simulink model "Propuesta_modelo_LIM"  (R2022b)
settings: Solver=VariableStepAuto  StartTime=0.0  StopTime=10.0  RelTol=1e-3
undefined symbols (not defined in the file or in its folder): mass, pole_length, Ref_velocity
libraries: slpidlib x2
settings Model: Creator=Javier  LastModifiedBy=Javier
settings DebuggingCC: UnconnectedInputMsg=warning  UnconnectedOutputMsg=warning  UnconnectedLineMsg=warning
settings ModelReferenceCC: EnableRefExpFcnMdlSchedulingChecks=on
settings RTWCC: DLArmComputeVersion=19.05

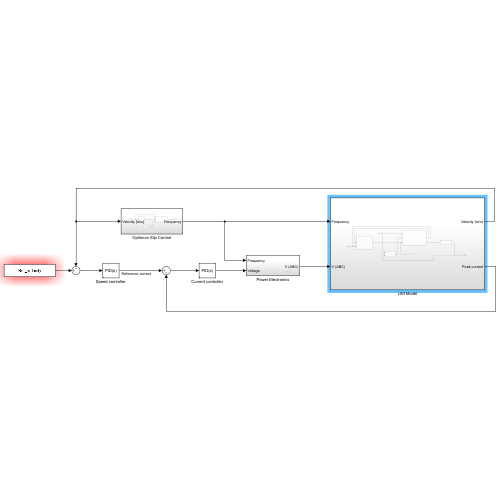
[thumbnail: Simulink's stored preview of the top-level diagram]
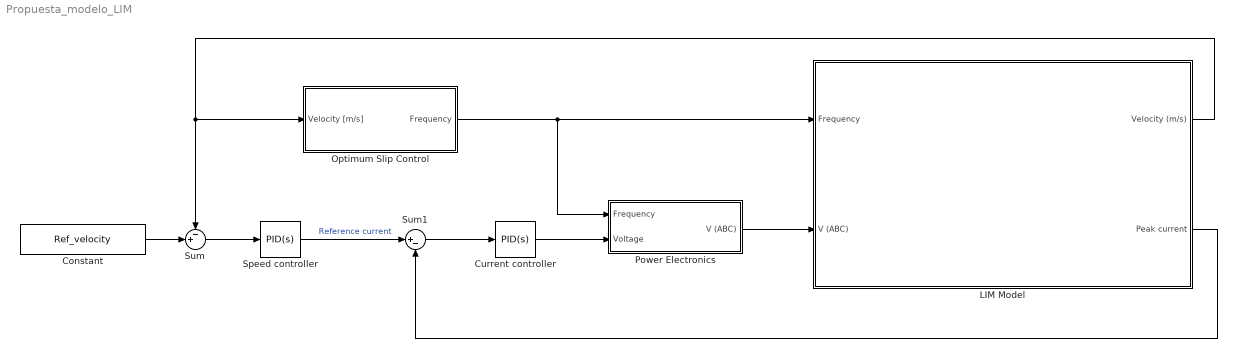
== system Propuesta_modelo_LIM ==
  Constant : Constant  Value=Ref_velocity
  Current controller : slpidlib/PID Controller  Controller=PID  Form=Parallel  TimeDomain=Continuous-time  UseExternalTs=off  SampleTime=-1  IntegratorMethod=Forward Euler  FilterMethod=Forward Euler  ControllerParametersSource=internal  P=1  I=1  UseKiTs=off  D=0  N=100  UseFilter=on  TunerSelectOption=Transfer Function Based (PID Tuner App)  InitialConditionSource=internal  InitialConditionForIntegrator=0  InitialConditionForFilter=0  DifferentiatorICPrevScaledInput=0  ExternalReset=none  TrackingMode=off  Kt=1  LimitOutput=off  SatLimitsSource=internal  UpperSaturationLimit=inf  LowerSaturationLimit=-inf  LinearizeAsGain=on  AntiWindupMode=none  Kb=1  LimitIntegrator=off  UpperIntegratorSaturationLimit=inf  LowerIntegratorSaturationLimit=-inf  POutMin=[]  POutMax=[]  IOutMin=[]  IOutMax=[]  DOutMin=[]  DOutMax=[]  NOutMin=[]  NOutMax=[]  SumOutMin=[]  SumOutMax=[]  SaturationOutMin=[]  SaturationOutMax=[]  PParamMin=[]  PParamMax=[]  IParamMin=[]  IParamMax=[]  DParamMin=[]  DParamMax=[]  NParamMin=[]  NParamMax=[]  KbParamMin=[]  KbParamMax=[]  KtParamMin=[]  KtParamMax=[]  KbOutMin=[]  KbOutMax=[]  KtOutMin=[]  KtOutMax=[]  IntegratorOutMin=[]  IntegratorOutMax=[]  FilterOutMin=[]  FilterOutMax=[]  SumI1OutMin=[]  SumI1OutMax=[]  SumI2OutMin=[]  SumI2OutMax=[]  SumI3OutMin=[]  SumI3OutMax=[]  SumI4OutMin=[]  SumI4OutMax=[]  SumDOutMin=[]  SumDOutMax=[]  DifferentiatorOutMin=[]  DifferentiatorOutMax=[]  FilterDiffOutCoefMin=[]  FilterDiffOutCoefMax=[]  ReciprocalOutMin=[]  ReciprocalOutMax=[]  SumDenOutMin=[]  SumDenOutMax=[]  SumNumOutMin=[]  SumNumOutMax=[]  DivideOutMin=[]  DivideOutMax=[]  UdiffTsProdOutMin=[]  UdiffTsProdOutMax=[]  NTsProdOutMin=[]  NTsProdOutMax=[]  UintegralTsProdOutMin=[]  UintegralTsProdOutMax=[]  UngainTsProdOutMin=[]  UngainTsProdOutMax=[]  ClampingZeroOutDataTypeStr=Inherit: Inherit via back propagation  ClampingZeroOutMin=[]  ClampingZeroOutMax=[]  FilterDenConstantOutDataTypeStr=Inherit: Inherit via back propagation  FilterDenConstantOutMin=[]  FilterDenConstantOutMax=[]  PCopyOutDataTypeStr=Inherit: Inherit via back propagation  PCopyOutMin=[]  PCopyOutMax=[]  NCopyOutDataTypeStr=Inherit: Inherit via back propagation  NCopyOutMin=[]  NCopyOutMax=[]  IntegratorContinuousStateAttributes=''  IntegratorStateMustResolveToSignalObject=off  IntegratorRTWStateStorageClass=Auto  FilterContinuousStateAttributes=''  FilterStateMustResolveToSignalObject=off  FilterRTWStateStorageClass=Auto  ParallelPVariant=InternalParameters  IdealPVariant=Disabled  IVariant=InternalParameters  DVariant=InternalParameters  IntegratorVariant=Continuous  SatVariant=Disabled  AWVariant=Passthrough  PCopyVariant=Disabled  TRVariant=Disabled  FdbkBlocksVariant=Forward  IdealPFdbkVariant=Disabled  SatFdbkVariant=Disabled  DerivativeFilterVariant=ContFilter  NVariant=InternalParameters  NCopyVariant=Disabled  FilterICVariant=InternalICsFilter  IntegratorICVariant=InternalICs  ExternalResetVariant=Disabled  TRSumVariant=Passthrough  SumFdbkVariant=Disabled  SumVariant=Sum_PID  TsampFilterVariant=InternalTs  TsampNgainVariant=Passthrough  TsampIntegralVariant=Passthrough  ExternalSaturationOutDataTypeStr=Inherit: Same as second input
  LIM Model : Subsystem
  Optimum Slip Control : Subsystem
  Power Electronics : Subsystem
  Speed controller : slpidlib/PID Controller  Controller=PID  Form=Parallel  TimeDomain=Continuous-time  UseExternalTs=off  SampleTime=-1  IntegratorMethod=Forward Euler  FilterMethod=Forward Euler  ControllerParametersSource=internal  P=1  I=1  UseKiTs=off  D=0  N=100  UseFilter=on  TunerSelectOption=Transfer Function Based (PID Tuner App)  InitialConditionSource=internal  InitialConditionForIntegrator=0  InitialConditionForFilter=0  DifferentiatorICPrevScaledInput=0  ExternalReset=none  TrackingMode=off  Kt=1  LimitOutput=off  SatLimitsSource=internal  UpperSaturationLimit=inf  LowerSaturationLimit=-inf  LinearizeAsGain=on  AntiWindupMode=none  Kb=1  LimitIntegrator=off  UpperIntegratorSaturationLimit=inf  LowerIntegratorSaturationLimit=-inf  POutMin=[]  POutMax=[]  IOutMin=[]  IOutMax=[]  DOutMin=[]  DOutMax=[]  NOutMin=[]  NOutMax=[]  SumOutMin=[]  SumOutMax=[]  SaturationOutMin=[]  SaturationOutMax=[]  PParamMin=[]  PParamMax=[]  IParamMin=[]  IParamMax=[]  DParamMin=[]  DParamMax=[]  NParamMin=[]  NParamMax=[]  KbParamMin=[]  KbParamMax=[]  KtParamMin=[]  KtParamMax=[]  KbOutMin=[]  KbOutMax=[]  KtOutMin=[]  KtOutMax=[]  IntegratorOutMin=[]  IntegratorOutMax=[]  FilterOutMin=[]  FilterOutMax=[]  SumI1OutMin=[]  SumI1OutMax=[]  SumI2OutMin=[]  SumI2OutMax=[]  SumI3OutMin=[]  SumI3OutMax=[]  SumI4OutMin=[]  SumI4OutMax=[]  SumDOutMin=[]  SumDOutMax=[]  DifferentiatorOutMin=[]  DifferentiatorOutMax=[]  FilterDiffOutCoefMin=[]  FilterDiffOutCoefMax=[]  ReciprocalOutMin=[]  ReciprocalOutMax=[]  SumDenOutMin=[]  SumDenOutMax=[]  SumNumOutMin=[]  SumNumOutMax=[]  DivideOutMin=[]  DivideOutMax=[]  UdiffTsProdOutMin=[]  UdiffTsProdOutMax=[]  NTsProdOutMin=[]  NTsProdOutMax=[]  UintegralTsProdOutMin=[]  UintegralTsProdOutMax=[]  UngainTsProdOutMin=[]  UngainTsProdOutMax=[]  ClampingZeroOutDataTypeStr=Inherit: Inherit via back propagation  ClampingZeroOutMin=[]  ClampingZeroOutMax=[]  FilterDenConstantOutDataTypeStr=Inherit: Inherit via back propagation  FilterDenConstantOutMin=[]  FilterDenConstantOutMax=[]  PCopyOutDataTypeStr=Inherit: Inherit via back propagation  PCopyOutMin=[]  PCopyOutMax=[]  NCopyOutDataTypeStr=Inherit: Inherit via back propagation  NCopyOutMin=[]  NCopyOutMax=[]  IntegratorContinuousStateAttributes=''  IntegratorStateMustResolveToSignalObject=off  IntegratorRTWStateStorageClass=Auto  FilterContinuousStateAttributes=''  FilterStateMustResolveToSignalObject=off  FilterRTWStateStorageClass=Auto  ParallelPVariant=InternalParameters  IdealPVariant=Disabled  IVariant=InternalParameters  DVariant=InternalParameters  IntegratorVariant=Continuous  SatVariant=Disabled  AWVariant=Passthrough  PCopyVariant=Disabled  TRVariant=Disabled  FdbkBlocksVariant=Forward  IdealPFdbkVariant=Disabled  SatFdbkVariant=Disabled  DerivativeFilterVariant=ContFilter  NVariant=InternalParameters  NCopyVariant=Disabled  FilterICVariant=InternalICsFilter  IntegratorICVariant=InternalICs  ExternalResetVariant=Disabled  TRSumVariant=Passthrough  SumFdbkVariant=Disabled  SumVariant=Sum_PID  TsampFilterVariant=InternalTs  TsampNgainVariant=Passthrough  TsampIntegralVariant=Passthrough  ExternalSaturationOutDataTypeStr=Inherit: Same as second input
  Sum : Sum  Inputs=-+|
  Sum1 : Sum  Inputs=|+-
  wires:
  Sum/1 -> Speed controller/1
  LIM Model/1(Velocity (m/s)) -> Sum/1, Optimum Slip Control/1(Velocity [m/s])
  Speed controller/1 -> Sum1/1  "Reference current"
  Current controller/1 -> Power Electronics/2(Voltage)
  Sum1/1 -> Current controller/1
  LIM Model/2(Peak current) -> Sum1/2
  Optimum Slip Control/1(Frequency) -> Power Electronics/1(Frequency), LIM Model/1(Frequency)
  Constant/1 -> Sum/2
  Power Electronics/1(V (ABC)) -> LIM Model/2(V (ABC))

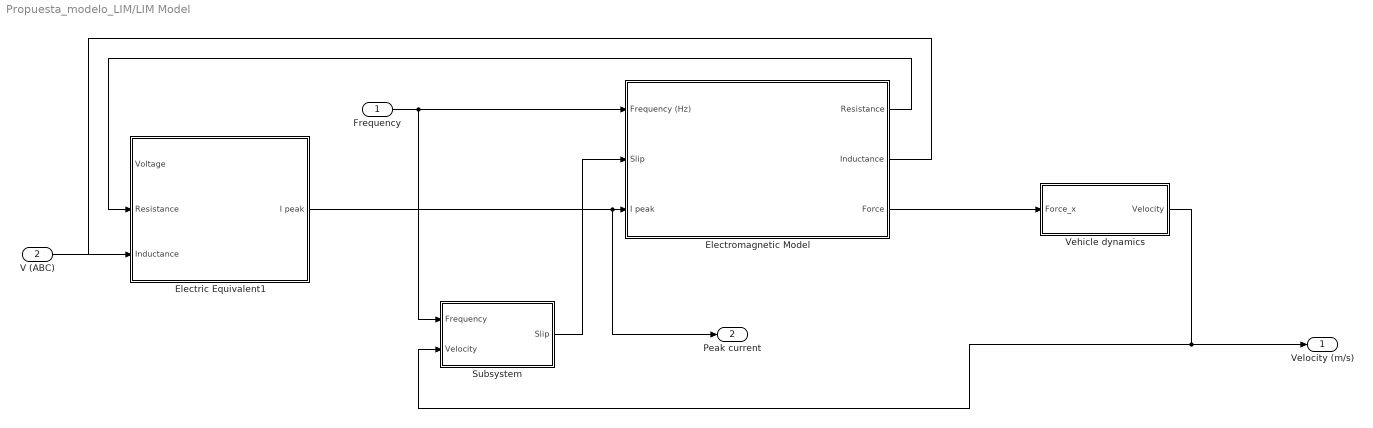
== system Propuesta_modelo_LIM/LIM Model ==
  Frequency : Inport
  V (ABC) : Inport  Port=2
  Electric Equivalent1 : Subsystem
  Electromagnetic Model : Subsystem
  Subsystem : Subsystem
  Vehicle dynamics : Subsystem
  Velocity (m/s) : Outport
  Peak current : Outport  Port=2
  wires:
  Subsystem/1(Slip) -> Electromagnetic Model/2(Slip)
  Vehicle dynamics/1(Velocity) -> Subsystem/2(Velocity), Velocity (m/s)/1
  Electric Equivalent1/1(I peak) -> Peak current/1, Electromagnetic Model/3(I peak)
  Electromagnetic Model/1(Resistance) -> Electric Equivalent1/2(Resistance)
  Electromagnetic Model/2(Inductance) -> Electric Equivalent1/3(Inductance)
  V (ABC)/1 -> ?
  Frequency/1 -> Electromagnetic Model/1(Frequency (Hz)), Subsystem/1(Frequency)
  Electromagnetic Model/3(Force) -> Vehicle dynamics/1(Force_x)

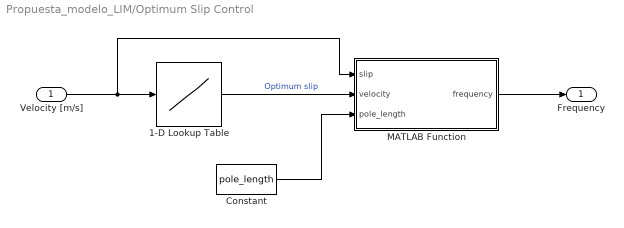
== system Propuesta_modelo_LIM/Optimum Slip Control ==
  Velocity [m/s] : Inport
  1-D Lookup Table : Lookup_n-D  NumberOfTableDimensions=1  BreakpointsForDimension1=[-5:5]  Table=tanh([-5:5])  InternalRulePriority=Speed  RndMeth=Simplest
  Constant : Constant  Value=pole_length
  MATLAB Function : MATLAB Function  TreatAsAtomicUnit=on
  Frequency : Outport
  wires:
  Velocity [m/s]/1 -> MATLAB Function/1(slip), 1-D Lookup Table/1
  1-D Lookup Table/1 -> MATLAB Function/2(velocity)  "Optimum slip"
  MATLAB Function/1(frequency) -> Frequency/1
  Constant/1 -> MATLAB Function/3(pole_length)

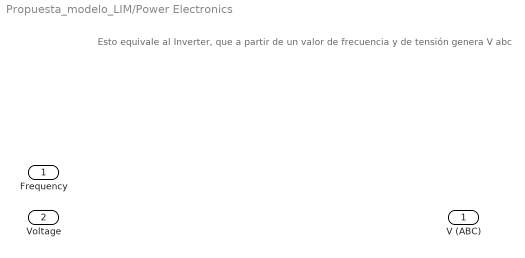
== system Propuesta_modelo_LIM/Power Electronics ==
  note: Esto equivale al Inverter, que a partir de un valor de frecuencia y de tensión genera V abc
  Frequency : Inport
  Voltage : Inport  Port=2
  V (ABC) : Outport

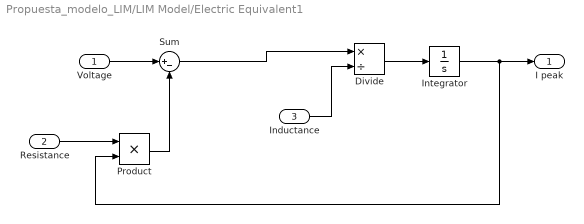
== system Propuesta_modelo_LIM/LIM Model/Electric Equivalent1 ==
  Voltage : Inport
  Resistance : Inport  Port=2
  Inductance : Inport  Port=3
  Divide : Product  Inputs=*/
  Integrator : Integrator
  Product : Product
  Sum : Sum  Inputs=|+-
  I peak : Outport
  wires:
  Voltage/1 -> Sum/1
  Integrator/1 -> Product/2, I peak/1
  Resistance/1 -> Product/1
  Product/1 -> Sum/2
  Divide/1 -> Integrator/1
  Sum/1 -> Divide/1
  Inductance/1 -> Divide/2

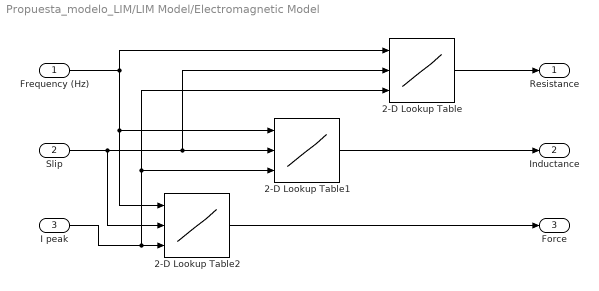
== system Propuesta_modelo_LIM/LIM Model/Electromagnetic Model ==
  Frequency (Hz) : Inport
  Slip : Inport  Port=2
  I peak : Inport  Port=3
  2-D Lookup Table : Lookup_n-D  NumberOfTableDimensions=3  BreakpointsForDimension1=[1:3]  BreakpointsForDimension2=[1:3]  InternalRulePriority=Speed  RndMeth=Simplest
      settings: InputPortMap=u0,u1,u2
  2-D Lookup Table1 : Lookup_n-D  NumberOfTableDimensions=3  BreakpointsForDimension1=[1:3]  BreakpointsForDimension2=[1:3]  InternalRulePriority=Speed  RndMeth=Simplest
      settings: InputPortMap=u0,u1,u2
  2-D Lookup Table2 : Lookup_n-D  NumberOfTableDimensions=3  BreakpointsForDimension1=[1:3]  BreakpointsForDimension2=[1:3]  InternalRulePriority=Speed  RndMeth=Simplest
      settings: InputPortMap=u0,u1,u2
  Resistance : Outport
  Inductance : Outport  Port=2
  Force : Outport  Port=3
  wires:
  2-D Lookup Table/1 -> Resistance/1
  2-D Lookup Table1/1 -> Inductance/1
  2-D Lookup Table2/1 -> Force/1
  I peak/1 -> 2-D Lookup Table1/3, 2-D Lookup Table/3, 2-D Lookup Table2/3
  Slip/1 -> 2-D Lookup Table2/2, 2-D Lookup Table/2, 2-D Lookup Table1/2
  Frequency (Hz)/1 -> 2-D Lookup Table/1, 2-D Lookup Table1/1, 2-D Lookup Table2/1

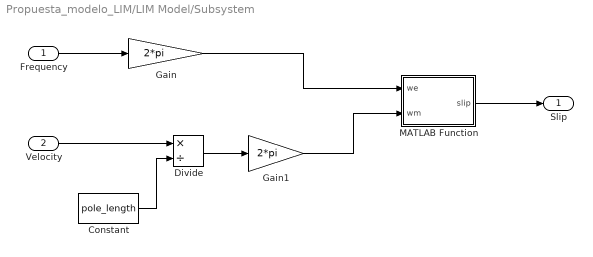
== system Propuesta_modelo_LIM/LIM Model/Subsystem ==
  Frequency : Inport
  Velocity : Inport  Port=2
  Constant : Constant  Value=pole_length
  Divide : Product  Inputs=*/
  Gain : Gain  Gain=2*pi
  Gain1 : Gain  Gain=2*pi
  MATLAB Function : MATLAB Function  TreatAsAtomicUnit=on
  Slip : Outport
  wires:
  Frequency/1 -> Gain/1
  Velocity/1 -> Divide/1
  Constant/1 -> Divide/2
  Divide/1 -> Gain1/1
  MATLAB Function/1(slip) -> Slip/1
  Gain/1 -> MATLAB Function/1(we)
  Gain1/1 -> MATLAB Function/2(wm)

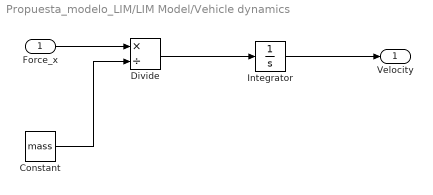
== system Propuesta_modelo_LIM/LIM Model/Vehicle dynamics ==
  Force_x : Inport
  Constant : Constant  Value=mass
  Divide : Product  Inputs=*/
  Integrator : Integrator
  Velocity : Outport
  wires:
  Force_x/1 -> Divide/1
  Divide/1 -> Integrator/1
  Integrator/1 -> Velocity/1
  Constant/1 -> Divide/2

== matlab function Propuesta_modelo_LIM/LIM Model/Subsystem/MATLAB Function ==
  data: we input; slip output; wm input
function slip = fcn(we,wm)

slip = (we-wm)/we;

== matlab function Propuesta_modelo_LIM/Optimum Slip Control/MATLAB Function ==
  data: slip input; velocity input; frequency output; pole_length input
function frequency = fcn(slip, velocity, pole_length)

ve = velocity / (1-slip);

frequency = (ve/pole_length)/(2*pi);
